simulink model "Vehicle_Model"  (R2019b)
settings: Solver=VariableStepAuto  StartTime=0.0  StopTime=20  RelTol=1e-3
libraries: mpcadaslib x1
settings Model: Creator=Yinglongli  LastModifiedBy=Yinglongli

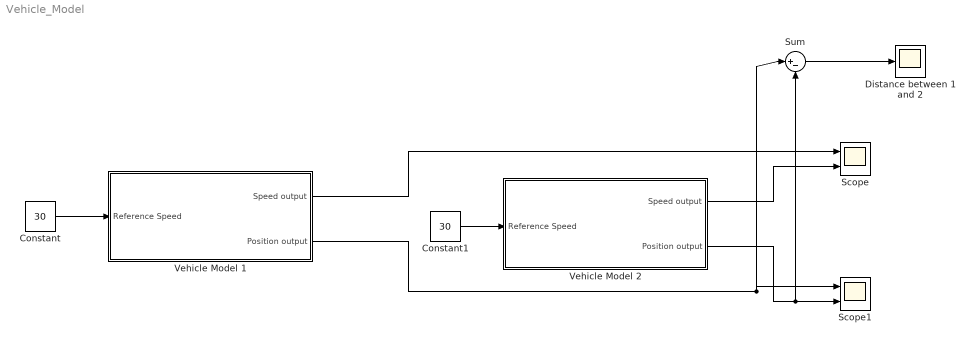
== system Vehicle_Model ==
  Constant : Constant  Value=30
  Constant1 : Constant  Value=30
  "Distance between 1 and 2 " : Scope
  Scope : Scope  NumInputPorts=2
  Scope1 : Scope  NumInputPorts=2
  Sum : Sum  Inputs=|+-
  Vehicle Model 1 : Subsystem  mask{pos=100, speed=10}
      mask prompts: pos "Initial Position"; speed "Initial Speed"
      mask TypeOptions pos: Initial Position/Value
      mask TypeOptions speed:
      | Initial Speed
      | /Value
  Vehicle Model 2 : Subsystem  mask{pos=50, speed=20}
      mask prompts: pos "Initial Position"; speed "Initial Speed"
      mask TypeOptions pos: Initial Position/Value
      mask TypeOptions speed:
      | Initial Speed
      | /Value
  wires:
  Constant/1 -> Vehicle Model 1/1("Reference Speed ")
  Vehicle Model 1/1("Speed output ") -> Scope/1
  Vehicle Model 1/2(Position output) -> Sum/1, Scope1/1
  Vehicle Model 2/1("Speed output ") -> Scope/2
  Vehicle Model 2/2(Position output) -> Sum/2, Scope1/2
  Constant1/1 -> Vehicle Model 2/1("Reference Speed ")
  Sum/1 -> "Distance between 1 and 2 "/1

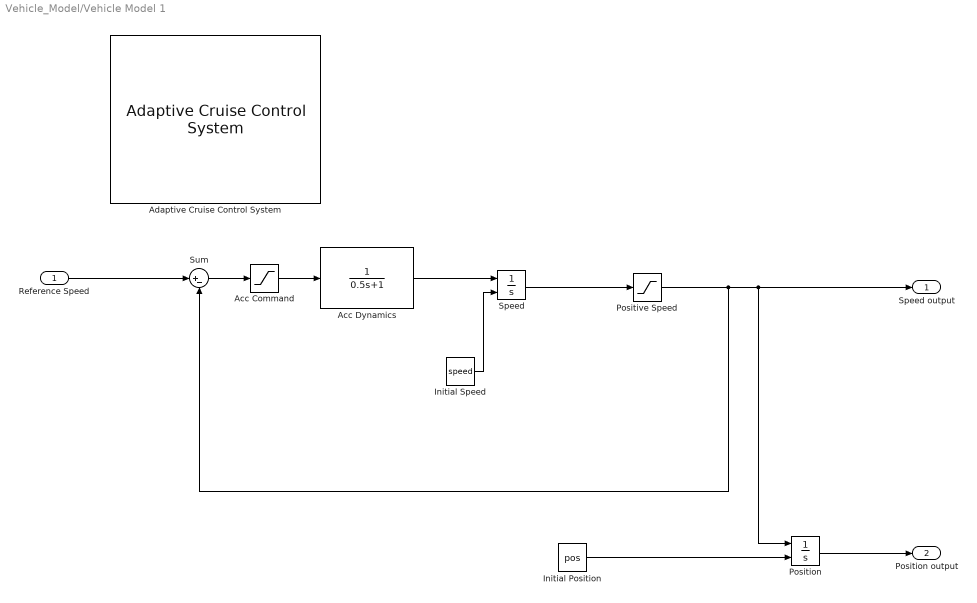
== system Vehicle_Model/Vehicle Model 1 ==
  "Reference Speed " : Inport
  Acc Command : Saturate  UpperLimit=2  LowerLimit=-3
  "Acc Dynamics " : TransferFcn  Denominator=[0.5 1]
  Adaptive Cruise Control System : mpcadaslib/Adaptive Cruise Control System  EgoModel=tf(1,[0.5,1,0])  InitialEgoVelocity=20  DefaultSpacing=10  MaxVelocity=50  MinAcceleration=-3  amin_ext=off  MaxAcceleration=2  amax_ext=off  Ts=0.1  PredictionHorizon=30  ControllerBehavior=0.5  suboptimal=off  maxiter=10  datatypeopt=double  optmode=off  trackmode=off
      settings: SourceProductName=Model Predictive Control Toolbox
  Initial Position : Constant  Value=pos
  "Initial Speed " : Constant  Value=speed
  Position : Integrator  InitialConditionSource=external
  Positive Speed : Saturate  UpperLimit=inf  LowerLimit=0
  Speed : Integrator  InitialConditionSource=external
  Sum : Sum  Inputs=|+-
  "Speed output " : Outport
  Position output : Outport  Port=2
  wires:
  Speed/1 -> Positive Speed/1
  Positive Speed/1 -> Sum/2, "Speed output "/1, Position/1
  Position/1 -> Position output/1
  Initial Position/1 -> Position/2
  "Acc Dynamics "/1 -> Speed/1
  "Reference Speed "/1 -> Sum/1
  "Initial Speed "/1 -> Speed/2
  Acc Command/1 -> "Acc Dynamics "/1
  Sum/1 -> Acc Command/1

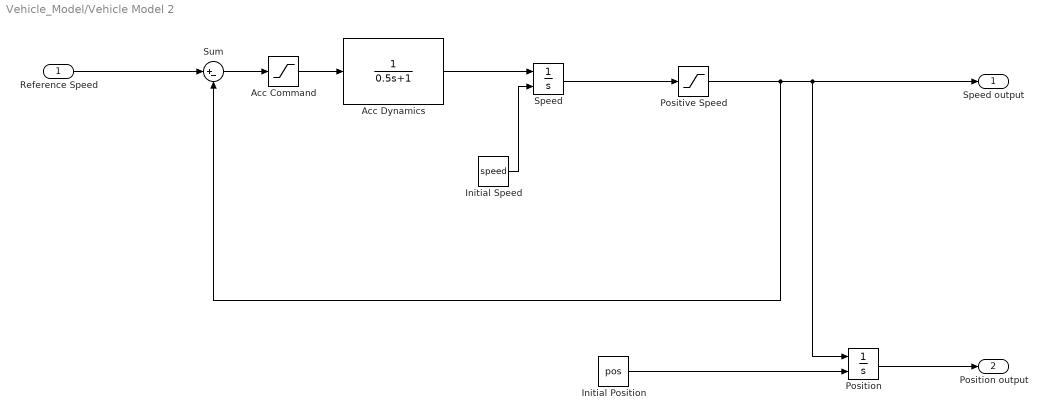
== system Vehicle_Model/Vehicle Model 2 ==
  "Reference Speed " : Inport
  Acc Command : Saturate  UpperLimit=2  LowerLimit=-3
  "Acc Dynamics " : TransferFcn  Denominator=[0.5 1]
  Initial Position : Constant  Value=pos
  "Initial Speed " : Constant  Value=speed
  Position : Integrator  InitialConditionSource=external
  Positive Speed : Saturate  UpperLimit=inf  LowerLimit=0
  Speed : Integrator  InitialConditionSource=external
  Sum : Sum  Inputs=|+-
  "Speed output " : Outport
  Position output : Outport  Port=2
  wires:
  Speed/1 -> Positive Speed/1
  Positive Speed/1 -> Sum/2, "Speed output "/1, Position/1
  Position/1 -> Position output/1
  Initial Position/1 -> Position/2
  "Acc Dynamics "/1 -> Speed/1
  "Reference Speed "/1 -> Sum/1
  "Initial Speed "/1 -> Speed/2
  Acc Command/1 -> "Acc Dynamics "/1
  Sum/1 -> Acc Command/1
